simulink model "mts"  (R2024a)
settings: Solver=FixedStepDiscrete  StartTime=0.0  StopTime=10  FixedStep=1  RelTol=1e-3
libraries: simulink x3
settings Model: Creator=batukar  LastModifiedBy=batukar
settings DebuggingCC: UnderspecifiedInitializationDetection=Classic

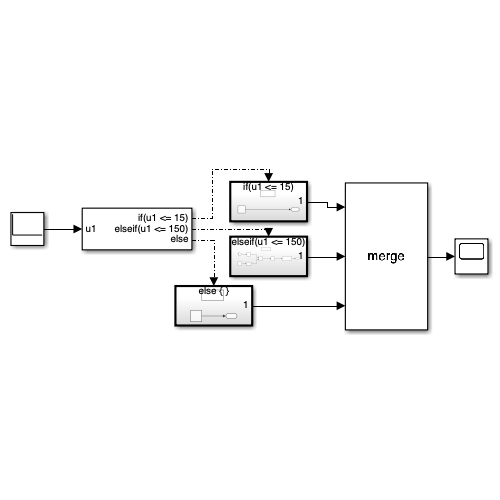
[thumbnail: Simulink's stored preview of the top-level diagram]
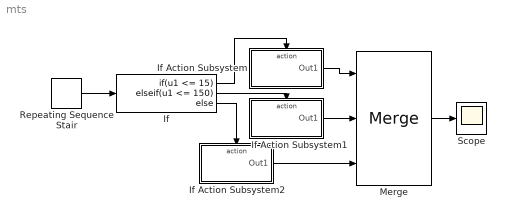
== system mts ==
  If : If  IfExpression=u1 <= 15  ElseIfExpressions=u1 <= 150
  If Action Subsystem : Subsystem  TreatAsAtomicUnit=on
  If Action Subsystem1 : Subsystem  TreatAsAtomicUnit=on
  If Action Subsystem2 : Subsystem  TreatAsAtomicUnit=on
  Merge : Merge  Inputs=3  InitialOutput=0
  Repeating Sequence Stair : simulink/Sources/Repeating Sequence Stair  OutValues=10  tsamp=1  OutMin=[]  OutMax=[]  OutDataTypeStr=double  OutputDataTypeScalingMode=double  OutDataType=fixdt(0,8)  ConRadixGroup=Best Precision: Vector-wise  OutScaling=2^-12
  Scope : Scope
  wires:
  Repeating Sequence Stair/1 -> If/1
  If/1 -> If Action Subsystem/Action
  If/2 -> If Action Subsystem1/Action
  If/3 -> If Action Subsystem2/Action
  If Action Subsystem/1(Out1) -> Merge/1
  If Action Subsystem2/1(Out1) -> Merge/3
  If Action Subsystem1/1(Out1) -> Merge/2
  Merge/1 -> Scope/1

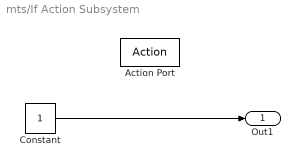
== system mts/If Action Subsystem ==
  Action Port : ActionPort  ActionPortLabel=if(u1 <= 15)
  Constant : Constant  SampleTime=-1  LockScale=on
  Out1 : Outport
  wires:
  Constant/1 -> Out1/1

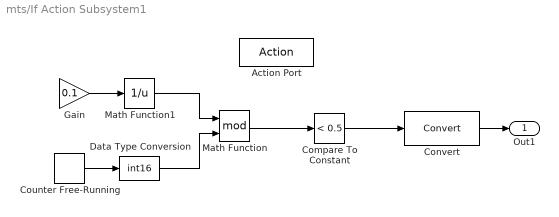
== system mts/If Action Subsystem1 ==
  Action Port : ActionPort  ActionPortLabel=elseif(u1 <= 150)
  Compare To Constant : simulink/Logic and Bit Operations/Compare To Constant  relop=<  const=0.5  OutDataTypeStr=boolean
  Convert : DataTypeConversion  SaturateOnIntegerOverflow=off  RndMeth=Floor
  Counter Free-Running : simulink/Sources/Counter Free-Running  NumBits=16  tsamp=-1
  Data Type Conversion : DataTypeConversion  OutDataTypeStr=int16  SaturateOnIntegerOverflow=off  RndMeth=Floor
  Gain : Gain  Gain=0.1  OutDataTypeStr=int16
      settings: AttributesFormatString=%<SampleTime>
  Math Function : Math  Operator=mod
  Math Function1 : Math  Operator=reciprocal
  Out1 : Outport
  wires:
  Counter Free-Running/1 -> Data Type Conversion/1
  Gain/1 -> Math Function1/1
  Compare To Constant/1 -> Convert/1
  Convert/1 -> Out1/1
  Data Type Conversion/1 -> Math Function/2
  Math Function1/1 -> Math Function/1
  Math Function/1 -> Compare To Constant/1

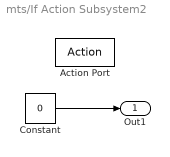
== system mts/If Action Subsystem2 ==
  Action Port : ActionPort  ActionPortLabel=else
  Constant : Constant  Value=0  VectorParams1D=off  SampleTime=-1
  Out1 : Outport  OutputWhenDisabled=reset  InitialOutput=0
  wires:
  Constant/1 -> Out1/1
